simulink model "FIR_Filter_Ref"  (R2020b)
settings: Solver=VariableStepAuto  StartTime=0.0  StopTime=10.0  RelTol=1e-3
settings Model: Creator=Shubham  LastModifiedBy=Shubham
settings DataIOCC: SaveOutput=off  SaveTime=off

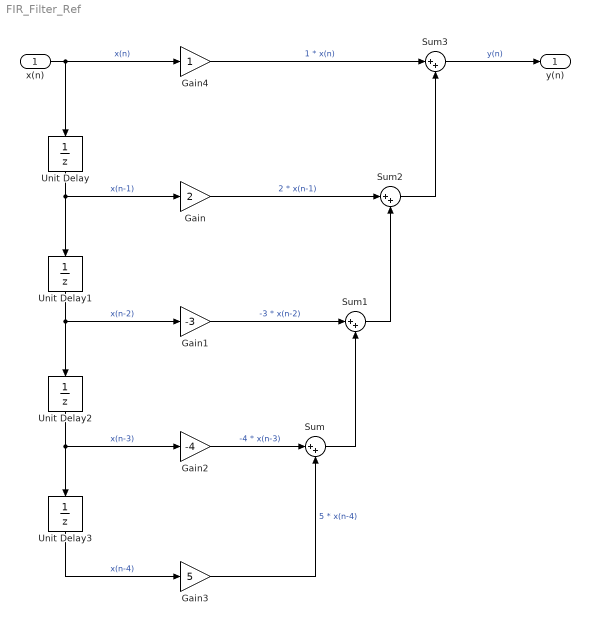
== system FIR_Filter_Ref ==
  x(n) : Inport  OutDataTypeStr=double  PortDimensions=1  SampleTime=0
  Gain : Gain  Gain=2
  Gain1 : Gain  Gain=-3
  Gain2 : Gain  Gain=-4
  Gain3 : Gain  Gain=5
  Gain4 : Gain
  Sum{,1..3} (4 alike) : Sum  Inputs=|++
  Unit Delay{,1..3} (4 alike) : UnitDelay  SampleTime=-1  HasFrameUpgradeWarning=on
  y(n) : Outport  OutDataTypeStr=double  PortDimensions=1  SampleTime=0
  wires:
  Gain1/1 -> Sum1/1  "-3 * x(n-2)"
  Unit Delay2/1 -> Unit Delay3/1, Gain2/1  "x(n-3)"
  Unit Delay/1 -> Unit Delay1/1, Gain/1  "x(n-1)"
  Gain2/1 -> Sum/1  "-4 * x(n-3)"
  Gain/1 -> Sum2/1  "2 * x(n-1)"
  Sum2/1 -> Sum3/2
  Sum1/1 -> Sum2/2
  Sum/1 -> Sum1/2
  Unit Delay3/1 -> Gain3/1  "x(n-4)"
  Gain3/1 -> Sum/2  "5 * x(n-4)"
  Gain4/1 -> Sum3/1  "1 * x(n)"
  Unit Delay1/1 -> Gain1/1, Unit Delay2/1  "x(n-2)"
  x(n)/1 -> Unit Delay/1, Gain4/1  "x(n)"
  Sum3/1 -> y(n)/1  "y(n)"
